simulink model "KTH_103002"  (Simulink 4.00)
settings: Solver=FixedStepDiscrete  StartTime=0.0  StopTime=5  RelTol=1e-3
values from neighbouring files (symbols this model uses):
  p2_1050 = [1.65 1.7 1.75 1.8 1.83 1.88 1.92 1.96 2.13 2.35 2.57 2.72 2.85 2.95]    [Comp1050_2.m]
  Pcomp_1050 = [690 790 880 1040 1160 1320 1580 1730 2970 5000 7960 9970 13200 16700]    [Comp1050_2.m]
  Qm_1050 = [2 2.5 3 4.5 5 6.5 8.5 10 20 35 55 65 85 100]    [Comp1050_2.m]
  T2_1050 = [99.2 103.5 107.2 110.7 111.8 112 111.7 100.4 116.5 131.5 136.4 147.4 149.6 155]    [Comp1050_2.m]
undefined symbols (not defined in the file or in its folder): conda, fan_cool, FC, fc_act, fc_blower_rec_H2, fc_blowera, fc_compressor, fc_condc, fc_coolstack, fc_current, fc_eqs, fc_evapcool, pump2, pump_cool, pump_re, radiator, vent
(part 2 of 2)

== system KTH_103002/PEM fuel cell system/Subsystem1/Anode init/Saturation pressure  anode humidifier ==
  note: Saturation pressure of water in the anode humidifier
      | NOTE: [bar]
      | Data from "Anlaggnings- och apparatteknik", Westerlund, T., Abo Akademi, Finland, 1998
  Anode humidifier temperature [C] : Constant  Value=FC.Lab.Temp.ah
  Anode humidifier temperature [C]1 : Constant  Value=FC.Lab.Temp.ah
  Constant : Constant  Value=11.78
  Constant1 : Constant  Value=99.64
  Constant2 : Constant  Value=230
  Math Function : Math  Operator=exp  OutputSignalType=auto
  Product : Product  Inputs=*/  Multiplication=Element-wise(.*)  SaturateOnIntegerOverflow=on
  Product1 : Product  Inputs=2  Multiplication=Element-wise(.*)  SaturateOnIntegerOverflow=on
  Sum : Sum  Inputs=|+-  SaturateOnIntegerOverflow=on
  Sum1 : Sum  Inputs=|++  SaturateOnIntegerOverflow=on
  psatah : Outport  Port=1
  tag scope: psatah=global
  wires:
  Anode humidifier temperature [C]/1 -> Sum/1
  Constant1/1 -> Sum/2
  Anode humidifier temperature [C]1/1 -> Sum1/1
  Constant2/1 -> Sum1/2
  Sum/1 -> Product/1
  Sum1/1 -> Product/2
  Constant/1 -> Product1/2
  Product/1 -> Product1/1
  Product1/1 -> Math Function/1
  Math Function/1 -> psatah/1, [psatah]

== system KTH_103002/PEM fuel cell system/Subsystem1/Anode init/Subsystem2 ==
  note: Activity of water vapor
  XWaI [-] : Inport  Port=1  LatchInput=off
  psatah [bar] : Inport  Port=2  LatchInput=off
  Constant : Constant  Value=FC.Lab.P.a
  Product : Product  Inputs=2  Multiplication=Element-wise(.*)  SaturateOnIntegerOverflow=on
  Product1 : Product  Inputs=*/  Multiplication=Element-wise(.*)  SaturateOnIntegerOverflow=on
  a : Outport  Port=1
  wires:
  XWaI [-]/1 -> Product/1
  Constant/1 -> Product/2
  Product/1 -> Product1/1
  psatah [bar]/1 -> Product1/2
  Product1/1 -> a/1

== system KTH_103002/PEM fuel cell system/Fuel cell stack, Heat Generation/Heat/Latent heat [W]/Heat of condensation ==
  note: Temperature in Celsius (C)
      | Tref=25 C
  note: 45.07E3 - 41.9*Tcell + 3.44E-3*Tcell^2 + 2.54E-6*Tcell^3 -8.98E-10*Tcell^4
  note: Heat of condensation [J/mol]
  Cell temperature [C] : Constant  Value=FC.Lab.Temp.cell
  Constant1 : Constant  Value=3.44E-3
  Constant2 : Constant  Value=45.07E3
  Constant3 : Constant  Value=41.9
  Constant4 : Constant  Value=2.54E-6
  Constant5 : Constant  Value=3
  Constant6 : Constant  Value=4
  Constant7 : Constant  Value=8.98E-10
  Display : Display
      settings: Format=short  Decimation=12
  Math Function : Math  Operator=square  OutputSignalType=auto
  Math Function1 : Math  Operator=pow  OutputSignalType=auto
  Math Function2 : Math  Operator=pow  OutputSignalType=auto
  Product{,1..3} (4 alike) : Product  Inputs=2  Multiplication=Element-wise(.*)  SaturateOnIntegerOverflow=on
  Sum : Sum  Inputs=|++  SaturateOnIntegerOverflow=on
  Sum1 : Sum  Inputs=|+-  SaturateOnIntegerOverflow=on
  Sum2 : Sum  Inputs=|++  SaturateOnIntegerOverflow=on
  Sum3 : Sum  Inputs=|+-  SaturateOnIntegerOverflow=on
  Hcond [J/mol] : Outport  Port=1
  wires:
  Constant3/1 -> Product/1
  Cell temperature [C]/1 -> Product/2, Math Function/1, Math Function1/1, Math Function2/1
  Product1/1 -> Sum/2
  Product/1 -> Sum1/2
  Constant2/1 -> Sum1/1
  Sum1/1 -> Sum/1
  Sum/1 -> Sum2/1
  Constant1/1 -> Product1/1
  Math Function/1 -> Product1/2
  Math Function1/1 -> Product2/2
  Constant4/1 -> Product2/1
  Product2/1 -> Sum2/2
  Sum2/1 -> Sum3/1
  Sum3/1 -> Hcond [J/mol]/1, Display/1
  Math Function2/1 -> Product3/2
  Product3/1 -> Sum3/2
  Constant7/1 -> Product3/1
  Constant5/1 -> Math Function1/2
  Constant6/1 -> Math Function2/2

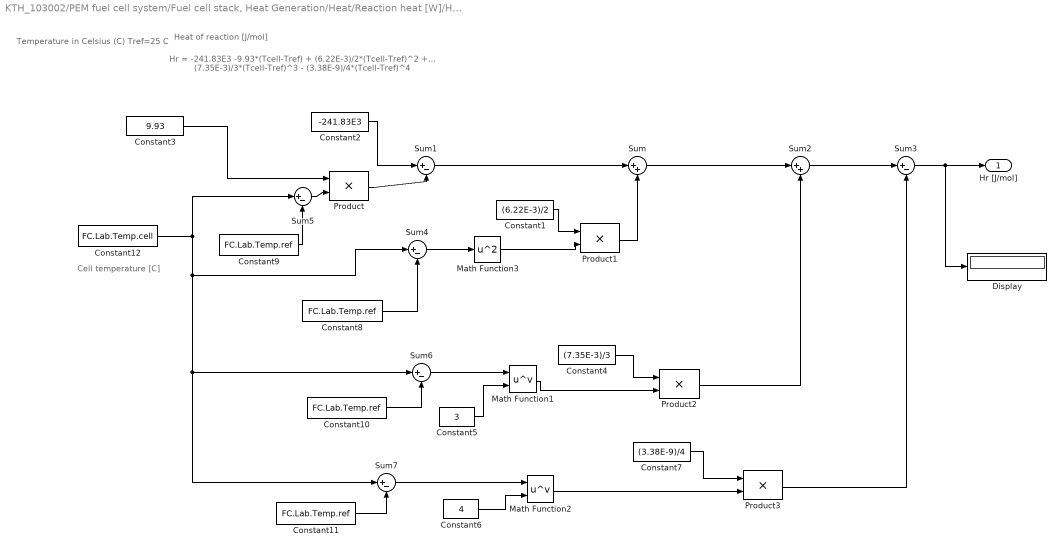
== system KTH_103002/PEM fuel cell system/Fuel cell stack, Heat Generation/Heat/Reaction heat [W]/Heat of reaction ==
  note: Temperature in Celsius (C)
      | Tref=25 C
  note: Hr = -241.83E3 -9.93*(Tcell-Tref) + (6.22E-3)/2*(Tcell-Tref)^2 +...
      |   (7.35E-3)/3*(Tcell-Tref)^3 - (3.38E-9)/4*(Tcell-Tref)^4
  note: Heat of reaction [J/mol]
  note: Cell temperature [C]
  Constant1 : Constant  Value=(6.22E-3)/2
  Constant{8..11} (4 alike) : Constant  Value=FC.Lab.Temp.ref
  Constant12 : Constant  Value=FC.Lab.Temp.cell
  Constant2 : Constant  Value=-241.83E3
  Constant3 : Constant  Value=9.93
  Constant4 : Constant  Value=(7.35E-3)/3
  Constant5 : Constant  Value=3
  Constant6 : Constant  Value=4
  Constant7 : Constant  Value=(3.38E-9)/4
  Display : Display
      settings: Format=short  Decimation=12
  Math Function1 : Math  Operator=pow  OutputSignalType=auto
  Math Function2 : Math  Operator=pow  OutputSignalType=auto
  Math Function3 : Math  Operator=square  OutputSignalType=auto
  Product{,1..3} (4 alike) : Product  Inputs=2  Multiplication=Element-wise(.*)  SaturateOnIntegerOverflow=on
  Sum : Sum  Inputs=|++  SaturateOnIntegerOverflow=on
  Sum{1,3..7} (6 alike) : Sum  Inputs=|+-  SaturateOnIntegerOverflow=on
  Sum2 : Sum  Inputs=|++  SaturateOnIntegerOverflow=on
  Hr [J/mol] : Outport  Port=1
  wires:
  Constant3/1 -> Product/1
  Product1/1 -> Sum/2
  Product/1 -> Sum1/2
  Constant2/1 -> Sum1/1
  Sum1/1 -> Sum/1
  Sum/1 -> Sum2/1
  Constant1/1 -> Product1/1
  Math Function1/1 -> Product2/2
  Constant4/1 -> Product2/1
  Product2/1 -> Sum2/2
  Sum2/1 -> Sum3/1
  Sum3/1 -> Hr [J/mol]/1, Display/1
  Math Function2/1 -> Product3/2
  Product3/1 -> Sum3/2
  Constant7/1 -> Product3/1
  Constant5/1 -> Math Function1/2
  Constant6/1 -> Math Function2/2
  Constant8/1 -> Sum4/2
  Sum5/1 -> Product/2
  Constant9/1 -> Sum5/2
  Sum4/1 -> Math Function3/1
  Math Function3/1 -> Product1/2
  Constant10/1 -> Sum6/2
  Sum6/1 -> Math Function1/1
  Constant11/1 -> Sum7/2
  Sum7/1 -> Math Function2/1
  Constant12/1 -> Sum5/1, Sum4/1, Sum6/1, Sum7/1

== system KTH_103002/PEM fuel cell system/Fuel cell stack, Heat Generation/Heat/Sensible heat [W]/Sensible heat in  ==
  note: Sensible heat in [W]
  note: Anode
  note: Cathode
  note: -------------------------------------------------------------------------------------------------------------------------------------------------------------------------------------------------------------------------------------------------------------------------------------------------------------------------------------------------------------------------------------------------------------------------------------------------------------------------------------------------------------------------------------------------------------------------------------------------------------------------------------------------------------------------------------------
  NinWa : Inport  Port=1  LatchInput=off
  NinHa : Inport  Port=2  LatchInput=off
  NinWc : Inport  Port=3  LatchInput=off
  NinO : Inport  Port=4  LatchInput=off
  NinN : Inport  Port=5  LatchInput=off
  "Enthalpy gaseous water, anode" : Subsystem
      settings: RTWFcnNameOpts=Auto  RTWFileNameOpts=Auto
  Enthalpy hydrogen in : Subsystem
      settings: RTWFcnNameOpts=Auto  RTWFileNameOpts=Auto
  Enthalpy nitrogen in : Subsystem
      settings: RTWFcnNameOpts=Auto  RTWFileNameOpts=Auto
  Enthalpy oxygen in : Subsystem
      settings: RTWFcnNameOpts=Auto  RTWFileNameOpts=Auto
  Product{,1..4} (5 alike) : Product  Inputs=2  Multiplication=Element-wise(.*)  SaturateOnIntegerOverflow=on
  Subsystem1 : Subsystem
      settings: RTWFcnNameOpts=Auto  RTWFileNameOpts=Auto
  Sum : Sum  Inputs=|++  SaturateOnIntegerOverflow=on
  Sum1 : Sum  Inputs=|++  SaturateOnIntegerOverflow=on
  Sum2 : Sum  Inputs=|++  SaturateOnIntegerOverflow=on
  sensina [W] : Outport  Port=1
  sensinc [W] : Outport  Port=2
  wires:
  NinHa/1 -> Product/1
  Enthalpy hydrogen in/1(h_Hin [J/mol]) -> Product/2
  Product/1 -> Sum/2
  NinWa/1 -> Product1/1
  Product1/1 -> Sum/1
  "Enthalpy gaseous water, anode"/1(h_Wgain [J/mol]) -> Product1/2
  NinWc/1 -> Product2/1
  Subsystem1/1(h_Wgcin [J/mol]) -> Product2/2
  Product2/1 -> Sum2/1
  NinO/1 -> Product3/1
  Enthalpy oxygen in/1(h_Oin [J/mol]) -> Product3/2
  Product3/1 -> Sum2/2
  Sum2/1 -> Sum1/1
  NinN/1 -> Product4/1
  Product4/1 -> Sum1/2
  Sum/1 -> sensina [W]/1
  Sum1/1 -> sensinc [W]/1
  Enthalpy nitrogen in/1(h_N [J/mol]) -> Product4/2

== system KTH_103002/PEM fuel cell system/Fuel cell stack, Heat Generation/Heat/Sensible heat [W]/Sensible heat out ==
  note: Sensible heat out [W]
  note: Anode
  note: Cathode
  note: -------------------------------------------------------------------------------------------------------------------------------------------------------------------------------------------------------------------------------------------------------------------------------------------------------------------------------------------------------------------------------------------------------------------------------------------------------------------------------------------------------------------------------------------------------------------------------------------------------------------------------------------------------------------------------------------
  note: Enthalpy gaseous water, cathode
  NoutWag : Inport  Port=1  LatchInput=off
  NoutHa : Inport  Port=2  LatchInput=off
  NoutWcg : Inport  Port=3  LatchInput=off
  NoutO : Inport  Port=4  LatchInput=off
  NoutN : Inport  Port=5  LatchInput=off
  NoutWcl : Inport  Port=6  LatchInput=off
  "Enthalpy gaseous water, anode" : Subsystem
      settings: RTWFcnNameOpts=Auto  RTWFileNameOpts=Auto
  Enthalpy hydrogen in : Subsystem
      settings: RTWFcnNameOpts=Auto  RTWFileNameOpts=Auto
  Enthalpy nitrogen out : Subsystem
      settings: RTWFcnNameOpts=Auto  RTWFileNameOpts=Auto
  Enthalpy oxygen out : Subsystem
      settings: RTWFcnNameOpts=Auto  RTWFileNameOpts=Auto
  Product{,1..5} (6 alike) : Product  Inputs=2  Multiplication=Element-wise(.*)  SaturateOnIntegerOverflow=on
  Subsystem1 : Subsystem
      settings: RTWFcnNameOpts=Auto  RTWFileNameOpts=Auto
  Subsystem2 : Subsystem
      settings: RTWFcnNameOpts=Auto  RTWFileNameOpts=Auto
  Sum{,1..3} (4 alike) : Sum  Inputs=|++  SaturateOnIntegerOverflow=on
  sensouta [W] : Outport  Port=1
  sensoutc [W] : Outport  Port=2
  wires:
  NoutHa/1 -> Product/1
  Enthalpy hydrogen in/1(h_Hout [J/mol]) -> Product/2
  Product/1 -> Sum/2
  NoutWag/1 -> Product1/1
  Product1/1 -> Sum/1
  "Enthalpy gaseous water, anode"/1(h_Wgaout [J/mol]) -> Product1/2
  NoutWcg/1 -> Product2/1
  Subsystem1/1(h_Wgcout [J/mol]) -> Product2/2
  Product2/1 -> Sum2/1
  NoutO/1 -> Product3/1
  Enthalpy oxygen out/1(h_Oout [J/mol]) -> Product3/2
  Product3/1 -> Sum2/2
  Sum2/1 -> Sum1/1
  NoutN/1 -> Product4/1
  Product4/1 -> Sum1/2
  Sum/1 -> sensouta [W]/1
  Enthalpy nitrogen out/1(h_N [J/mol]) -> Product4/2
  Sum1/1 -> Sum3/1
  Sum3/1 -> sensoutc [W]/1
  Subsystem2/1(h_Wl [J/mol]) -> Product5/2
  Product5/1 -> Sum3/2
  NoutWcl/1 -> Product5/1

== system KTH_103002/PEM fuel cell system/Humidifiers/Evapcooler/Ambient air/Humidity in air ==
  note: Humidity in air
  psat_air : Inport  Port=1  LatchInput=off
  Constant : Constant  Value=FC.Const.MW
  Constant1 : Constant  Value=FC.Lab.Stoich.RHo
  Constant2 : Constant  Value=FC.Const.Mair
  Constant3 : Constant  Value=FC.Lab.P.amb
  Constant4 : Constant  Value=100
  Constant6 : Constant  Value=FC.Lab.Stoich.RHo
  Constant7 : Constant  Value=100
  Display{,1..6} (7 alike) : Display
      settings: Format=short
  Product : Product  Inputs=*/  Multiplication=Element-wise(.*)  SaturateOnIntegerOverflow=on
  Product1 : Product  Inputs=*/  Multiplication=Element-wise(.*)  SaturateOnIntegerOverflow=on
  Product2 : Product  Inputs=3  Multiplication=Element-wise(.*)  SaturateOnIntegerOverflow=on
  Product3 : Product  Inputs=*/  Multiplication=Element-wise(.*)  SaturateOnIntegerOverflow=on
  Product4 : Product  Inputs=2  Multiplication=Element-wise(.*)  SaturateOnIntegerOverflow=on
  Product5 : Product  Inputs=/*  Multiplication=Element-wise(.*)  SaturateOnIntegerOverflow=on
  Sum : Sum  Inputs=|+-  SaturateOnIntegerOverflow=on
  wires:
  Constant/1 -> Product/1
  Constant2/1 -> Product/2
  Constant1/1 -> Product1/1
  Constant4/1 -> Product1/2
  psat_air/1 -> Product2/1, Product4/2
  Product1/1 -> Product2/3, Display4/1
  Product/1 -> Product2/2, Display3/1
  Constant6/1 -> Product3/1
  Constant7/1 -> Product3/2
  Constant3/1 -> Sum/1, Display6/1
  Product3/1 -> Sum/2
  Sum/1 -> Product4/1, Display5/1
  Product2/1 -> Product5/2, Display2/1
  Product4/1 -> Product5/1, Display1/1
  Product5/1 -> Display/1

== system KTH_103002/PEM fuel cell system/Humidifiers/Evapcooler/Ambient air/Saturation pressure ==
  note: Saturation pressure of water in the ambient air
      | NOTE: [bar]
      | Data from "Anlaggnings- och apparatteknik", Westerlund, T., Abo Akademi, Finland, 1998
  Ambient temperature [C] : Constant  Value=FC.Lab.Temp.amb
  Ambient temperature [C]1 : Constant  Value=FC.Lab.Temp.amb
  Constant : Constant  Value=11.78
  Constant1 : Constant  Value=99.64
  Constant2 : Constant  Value=230
  Display : Display
      settings: Format=short
  Math Function : Math  Operator=exp  OutputSignalType=auto
  Product : Product  Inputs=*/  Multiplication=Element-wise(.*)  SaturateOnIntegerOverflow=on
  Product1 : Product  Inputs=2  Multiplication=Element-wise(.*)  SaturateOnIntegerOverflow=on
  Sum : Sum  Inputs=|+-  SaturateOnIntegerOverflow=on
  Sum1 : Sum  Inputs=|++  SaturateOnIntegerOverflow=on
  psat_air : Outport  Port=1
  tag scope: psat_air=global
  wires:
  Ambient temperature [C]/1 -> Sum/1
  Constant1/1 -> Sum/2
  Ambient temperature [C]1/1 -> Sum1/1
  Constant2/1 -> Sum1/2
  Sum/1 -> Product/1
  Sum1/1 -> Product/2
  Constant/1 -> Product1/2
  Product/1 -> Product1/1
  Product1/1 -> Math Function/1
  Math Function/1 -> Display/1, psat_air/1, [psat_air]

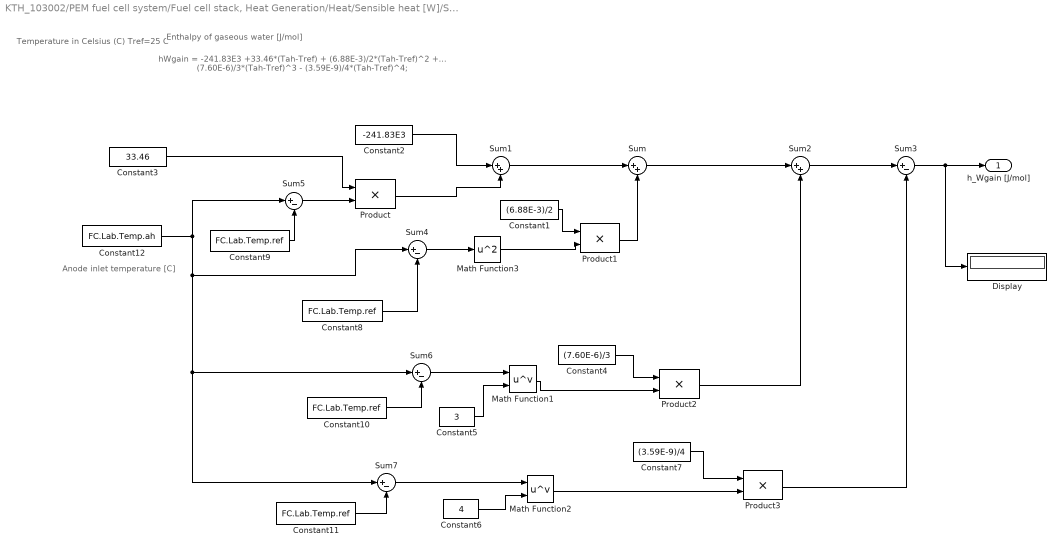
== system KTH_103002/PEM fuel cell system/Fuel cell stack, Heat Generation/Heat/Sensible heat [W]/Sensible heat in /Enthalpy gaseous water, anode ==
  note: Temperature in Celsius (C)
      | Tref=25 C
  note: hWgain = -241.83E3 +33.46*(Tah-Tref) + (6.88E-3)/2*(Tah-Tref)^2 +...
      |    (7.60E-6)/3*(Tah-Tref)^3 - (3.59E-9)/4*(Tah-Tref)^4;
  note: Enthalpy of gaseous water [J/mol]
  note: Anode inlet temperature [C]
  Constant1 : Constant  Value=(6.88E-3)/2
  Constant{8..11} (4 alike) : Constant  Value=FC.Lab.Temp.ref
  Constant12 : Constant  Value=FC.Lab.Temp.ah
  Constant2 : Constant  Value=-241.83E3
  Constant3 : Constant  Value=33.46
  Constant4 : Constant  Value=(7.60E-6)/3
  Constant5 : Constant  Value=3
  Constant6 : Constant  Value=4
  Constant7 : Constant  Value=(3.59E-9)/4
  Display : Display
      settings: Format=short  Decimation=12
  Math Function1 : Math  Operator=pow  OutputSignalType=auto
  Math Function2 : Math  Operator=pow  OutputSignalType=auto
  Math Function3 : Math  Operator=square  OutputSignalType=auto
  Product{,1..3} (4 alike) : Product  Inputs=2  Multiplication=Element-wise(.*)  SaturateOnIntegerOverflow=on
  Sum : Sum  Inputs=|++  SaturateOnIntegerOverflow=on
  Sum1 : Sum  Inputs=|++  SaturateOnIntegerOverflow=on
  Sum2 : Sum  Inputs=|++  SaturateOnIntegerOverflow=on
  Sum{3..7} (5 alike) : Sum  Inputs=|+-  SaturateOnIntegerOverflow=on
  h_Wgain [J/mol] : Outport  Port=1
  wires:
  Constant3/1 -> Product/1
  Product1/1 -> Sum/2
  Sum/1 -> Sum2/1
  Constant1/1 -> Product1/1
  Math Function1/1 -> Product2/2
  Constant4/1 -> Product2/1
  Product2/1 -> Sum2/2
  Sum2/1 -> Sum3/1
  Sum3/1 -> h_Wgain [J/mol]/1, Display/1
  Math Function2/1 -> Product3/2
  Product3/1 -> Sum3/2
  Constant7/1 -> Product3/1
  Constant5/1 -> Math Function1/2
  Constant6/1 -> Math Function2/2
  Constant8/1 -> Sum4/2
  Sum5/1 -> Product/2
  Constant9/1 -> Sum5/2
  Sum4/1 -> Math Function3/1
  Math Function3/1 -> Product1/2
  Constant10/1 -> Sum6/2
  Sum6/1 -> Math Function1/1
  Constant11/1 -> Sum7/2
  Sum7/1 -> Math Function2/1
  Constant12/1 -> Sum5/1, Sum4/1, Sum6/1, Sum7/1
  Product/1 -> Sum1/2
  Sum1/1 -> Sum/1
  Constant2/1 -> Sum1/1

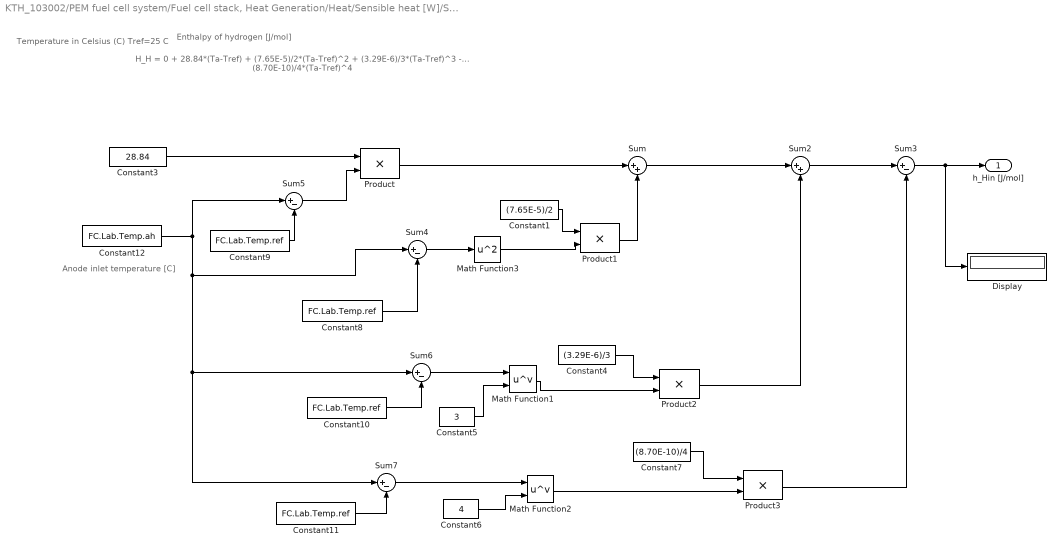
== system KTH_103002/PEM fuel cell system/Fuel cell stack, Heat Generation/Heat/Sensible heat [W]/Sensible heat in /Enthalpy hydrogen in ==
  note: Temperature in Celsius (C)
      | Tref=25 C
  note: H_H = 0 + 28.84*(Ta-Tref) + (7.65E-5)/2*(Ta-Tref)^2 + (3.29E-6)/3*(Ta-Tref)^3 -...
      |    (8.70E-10)/4*(Ta-Tref)^4
  note: Enthalpy of hydrogen [J/mol]
  note: Anode inlet temperature [C]
  Constant1 : Constant  Value=(7.65E-5)/2
  Constant{8..11} (4 alike) : Constant  Value=FC.Lab.Temp.ref
  Constant12 : Constant  Value=FC.Lab.Temp.ah
  Constant3 : Constant  Value=28.84
  Constant4 : Constant  Value=(3.29E-6)/3
  Constant5 : Constant  Value=3
  Constant6 : Constant  Value=4
  Constant7 : Constant  Value=(8.70E-10)/4
  Display : Display
      settings: Format=short  Decimation=12
  Math Function1 : Math  Operator=pow  OutputSignalType=auto
  Math Function2 : Math  Operator=pow  OutputSignalType=auto
  Math Function3 : Math  Operator=square  OutputSignalType=auto
  Product{,1..3} (4 alike) : Product  Inputs=2  Multiplication=Element-wise(.*)  SaturateOnIntegerOverflow=on
  Sum : Sum  Inputs=|++  SaturateOnIntegerOverflow=on
  Sum2 : Sum  Inputs=|++  SaturateOnIntegerOverflow=on
  Sum{3..7} (5 alike) : Sum  Inputs=|+-  SaturateOnIntegerOverflow=on
  h_Hin [J/mol] : Outport  Port=1
  wires:
  Constant3/1 -> Product/1
  Product1/1 -> Sum/2
  Sum/1 -> Sum2/1
  Constant1/1 -> Product1/1
  Math Function1/1 -> Product2/2
  Constant4/1 -> Product2/1
  Product2/1 -> Sum2/2
  Sum2/1 -> Sum3/1
  Sum3/1 -> h_Hin [J/mol]/1, Display/1
  Math Function2/1 -> Product3/2
  Product3/1 -> Sum3/2
  Constant7/1 -> Product3/1
  Constant5/1 -> Math Function1/2
  Constant6/1 -> Math Function2/2
  Constant8/1 -> Sum4/2
  Sum5/1 -> Product/2
  Constant9/1 -> Sum5/2
  Sum4/1 -> Math Function3/1
  Math Function3/1 -> Product1/2
  Constant10/1 -> Sum6/2
  Sum6/1 -> Math Function1/1
  Constant11/1 -> Sum7/2
  Sum7/1 -> Math Function2/1
  Constant12/1 -> Sum5/1, Sum4/1, Sum6/1, Sum7/1
  Product/1 -> Sum/1

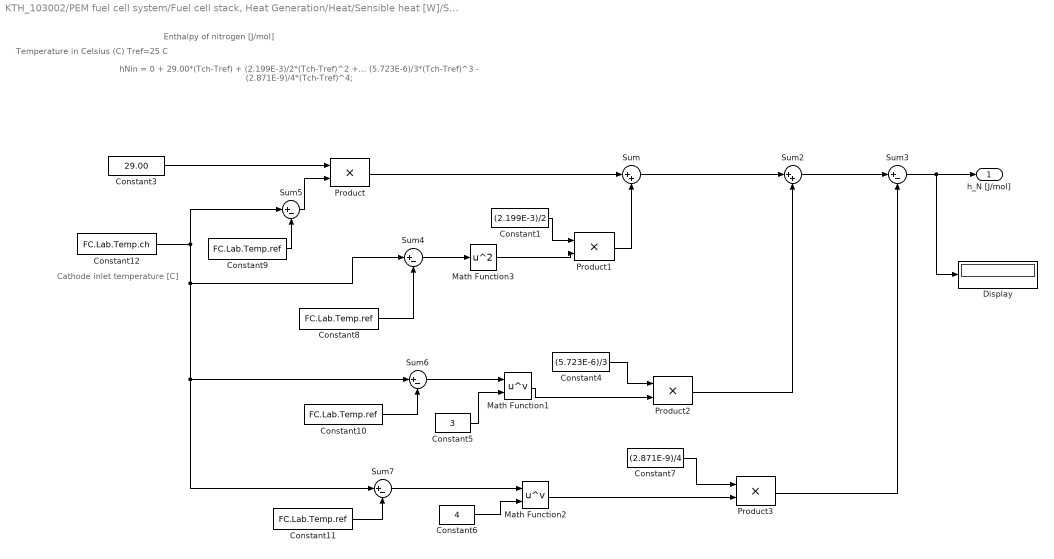
== system KTH_103002/PEM fuel cell system/Fuel cell stack, Heat Generation/Heat/Sensible heat [W]/Sensible heat in /Enthalpy nitrogen in ==
  note: Temperature in Celsius (C)
      | Tref=25 C
  note: hNin = 0 + 29.00*(Tch-Tref) + (2.199E-3)/2*(Tch-Tref)^2 +...
      |    (5.723E-6)/3*(Tch-Tref)^3 - (2.871E-9)/4*(Tch-Tref)^4;
  note: Enthalpy of nitrogen [J/mol]
  note: Cathode inlet temperature [C]
  Constant1 : Constant  Value=(2.199E-3)/2
  Constant{8..11} (4 alike) : Constant  Value=FC.Lab.Temp.ref
  Constant12 : Constant  Value=FC.Lab.Temp.ch
  Constant3 : Constant  Value=29.00
  Constant4 : Constant  Value=(5.723E-6)/3
  Constant5 : Constant  Value=3
  Constant6 : Constant  Value=4
  Constant7 : Constant  Value=(2.871E-9)/4
  Display : Display
      settings: Format=short  Decimation=12
  Math Function1 : Math  Operator=pow  OutputSignalType=auto
  Math Function2 : Math  Operator=pow  OutputSignalType=auto
  Math Function3 : Math  Operator=square  OutputSignalType=auto
  Product{,1..3} (4 alike) : Product  Inputs=2  Multiplication=Element-wise(.*)  SaturateOnIntegerOverflow=on
  Sum : Sum  Inputs=|++  SaturateOnIntegerOverflow=on
  Sum2 : Sum  Inputs=|++  SaturateOnIntegerOverflow=on
  Sum{3..7} (5 alike) : Sum  Inputs=|+-  SaturateOnIntegerOverflow=on
  h_N [J/mol] : Outport  Port=1
  wires:
  Constant3/1 -> Product/1
  Product1/1 -> Sum/2
  Product/1 -> Sum/1
  Sum/1 -> Sum2/1
  Constant1/1 -> Product1/1
  Math Function1/1 -> Product2/2
  Constant4/1 -> Product2/1
  Product2/1 -> Sum2/2
  Sum2/1 -> Sum3/1
  Sum3/1 -> h_N [J/mol]/1, Display/1
  Math Function2/1 -> Product3/2
  Product3/1 -> Sum3/2
  Constant7/1 -> Product3/1
  Constant5/1 -> Math Function1/2
  Constant6/1 -> Math Function2/2
  Constant8/1 -> Sum4/2
  Sum5/1 -> Product/2
  Constant9/1 -> Sum5/2
  Sum4/1 -> Math Function3/1
  Math Function3/1 -> Product1/2
  Constant10/1 -> Sum6/2
  Sum6/1 -> Math Function1/1
  Constant11/1 -> Sum7/2
  Sum7/1 -> Math Function2/1
  Constant12/1 -> Sum5/1, Sum4/1, Sum6/1, Sum7/1

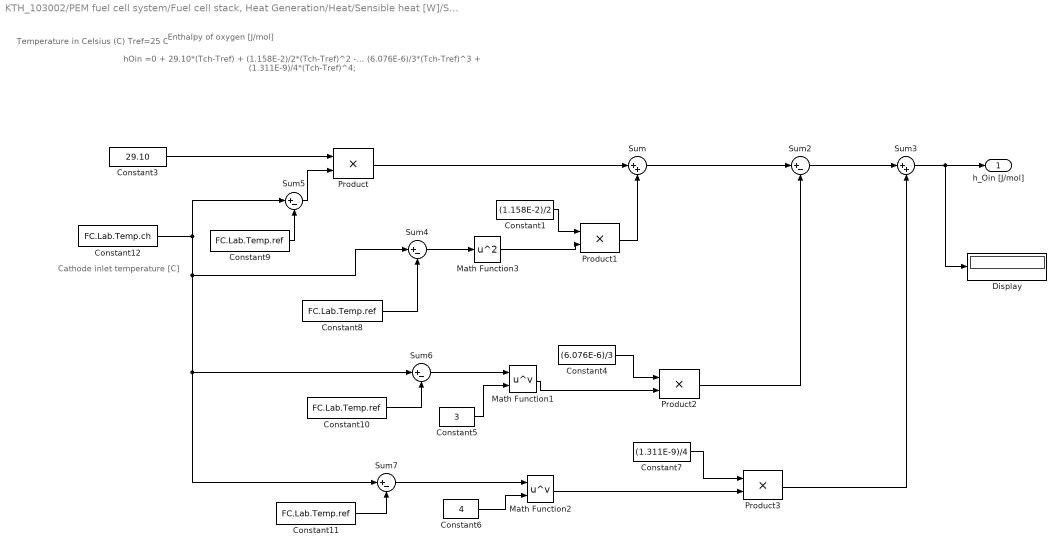
== system KTH_103002/PEM fuel cell system/Fuel cell stack, Heat Generation/Heat/Sensible heat [W]/Sensible heat in /Enthalpy oxygen in ==
  note: Temperature in Celsius (C)
      | Tref=25 C
  note: hOin =0 + 29.10*(Tch-Tref) + (1.158E-2)/2*(Tch-Tref)^2 -...
      |    (6.076E-6)/3*(Tch-Tref)^3 + (1.311E-9)/4*(Tch-Tref)^4;
  note: Enthalpy of oxygen [J/mol]
  note: Cathode inlet temperature [C]
  Constant1 : Constant  Value=(1.158E-2)/2
  Constant{8..11} (4 alike) : Constant  Value=FC.Lab.Temp.ref
  Constant12 : Constant  Value=FC.Lab.Temp.ch
  Constant3 : Constant  Value=29.10
  Constant4 : Constant  Value=(6.076E-6)/3
  Constant5 : Constant  Value=3
  Constant6 : Constant  Value=4
  Constant7 : Constant  Value=(1.311E-9)/4
  Display : Display
      settings: Format=short  Decimation=12
  Math Function1 : Math  Operator=pow  OutputSignalType=auto
  Math Function2 : Math  Operator=pow  OutputSignalType=auto
  Math Function3 : Math  Operator=square  OutputSignalType=auto
  Product{,1..3} (4 alike) : Product  Inputs=2  Multiplication=Element-wise(.*)  SaturateOnIntegerOverflow=on
  Sum : Sum  Inputs=|++  SaturateOnIntegerOverflow=on
  Sum{2,4..7} (5 alike) : Sum  Inputs=|+-  SaturateOnIntegerOverflow=on
  Sum3 : Sum  Inputs=|++  SaturateOnIntegerOverflow=on
  h_Oin [J/mol] : Outport  Port=1
  wires:
  Constant3/1 -> Product/1
  Product1/1 -> Sum/2
  Product/1 -> Sum/1
  Sum/1 -> Sum2/1
  Constant1/1 -> Product1/1
  Math Function1/1 -> Product2/2
  Constant4/1 -> Product2/1
  Product2/1 -> Sum2/2
  Sum2/1 -> Sum3/1
  Sum3/1 -> h_Oin [J/mol]/1, Display/1
  Math Function2/1 -> Product3/2
  Product3/1 -> Sum3/2
  Constant7/1 -> Product3/1
  Constant5/1 -> Math Function1/2
  Constant6/1 -> Math Function2/2
  Constant8/1 -> Sum4/2
  Sum5/1 -> Product/2
  Constant9/1 -> Sum5/2
  Sum4/1 -> Math Function3/1
  Math Function3/1 -> Product1/2
  Constant10/1 -> Sum6/2
  Sum6/1 -> Math Function1/1
  Constant11/1 -> Sum7/2
  Sum7/1 -> Math Function2/1
  Constant12/1 -> Sum5/1, Sum4/1, Sum6/1, Sum7/1

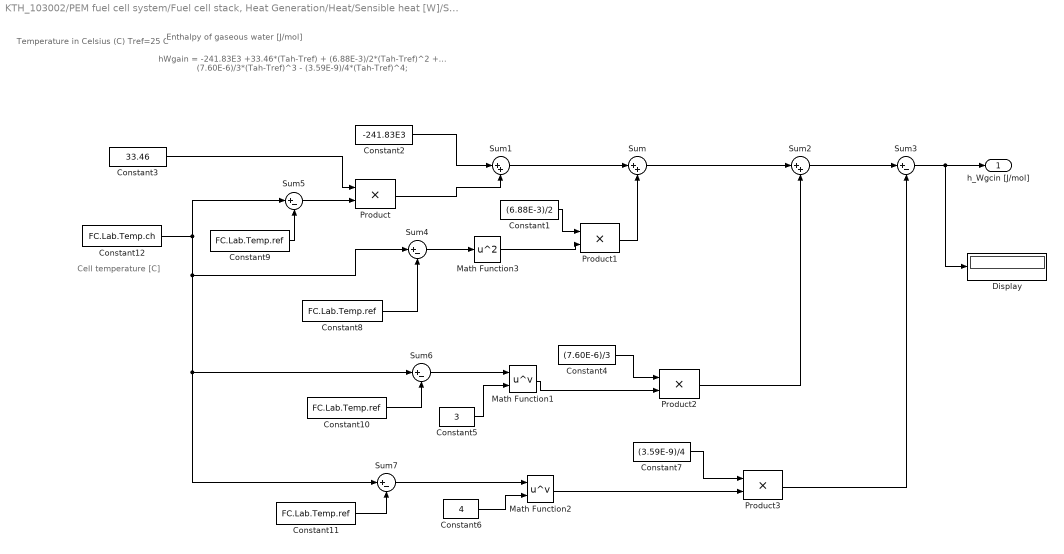
== system KTH_103002/PEM fuel cell system/Fuel cell stack, Heat Generation/Heat/Sensible heat [W]/Sensible heat in /Subsystem1 ==
  note: Temperature in Celsius (C)
      | Tref=25 C
  note: hWgain = -241.83E3 +33.46*(Tah-Tref) + (6.88E-3)/2*(Tah-Tref)^2 +...
      |    (7.60E-6)/3*(Tah-Tref)^3 - (3.59E-9)/4*(Tah-Tref)^4;
  note: Enthalpy of gaseous water [J/mol]
  note: Cell temperature [C]
  Constant1 : Constant  Value=(6.88E-3)/2
  Constant{8..11} (4 alike) : Constant  Value=FC.Lab.Temp.ref
  Constant12 : Constant  Value=FC.Lab.Temp.ch
  Constant2 : Constant  Value=-241.83E3
  Constant3 : Constant  Value=33.46
  Constant4 : Constant  Value=(7.60E-6)/3
  Constant5 : Constant  Value=3
  Constant6 : Constant  Value=4
  Constant7 : Constant  Value=(3.59E-9)/4
  Display : Display
      settings: Format=short  Decimation=12
  Math Function1 : Math  Operator=pow  OutputSignalType=auto
  Math Function2 : Math  Operator=pow  OutputSignalType=auto
  Math Function3 : Math  Operator=square  OutputSignalType=auto
  Product{,1..3} (4 alike) : Product  Inputs=2  Multiplication=Element-wise(.*)  SaturateOnIntegerOverflow=on
  Sum : Sum  Inputs=|++  SaturateOnIntegerOverflow=on
  Sum1 : Sum  Inputs=|++  SaturateOnIntegerOverflow=on
  Sum2 : Sum  Inputs=|++  SaturateOnIntegerOverflow=on
  Sum{3..7} (5 alike) : Sum  Inputs=|+-  SaturateOnIntegerOverflow=on
  h_Wgcin [J/mol] : Outport  Port=1
  wires:
  Constant3/1 -> Product/1
  Product1/1 -> Sum/2
  Sum/1 -> Sum2/1
  Constant1/1 -> Product1/1
  Math Function1/1 -> Product2/2
  Constant4/1 -> Product2/1
  Product2/1 -> Sum2/2
  Sum2/1 -> Sum3/1
  Sum3/1 -> h_Wgcin [J/mol]/1, Display/1
  Math Function2/1 -> Product3/2
  Product3/1 -> Sum3/2
  Constant7/1 -> Product3/1
  Constant5/1 -> Math Function1/2
  Constant6/1 -> Math Function2/2
  Constant8/1 -> Sum4/2
  Sum5/1 -> Product/2
  Constant9/1 -> Sum5/2
  Sum4/1 -> Math Function3/1
  Math Function3/1 -> Product1/2
  Constant10/1 -> Sum6/2
  Sum6/1 -> Math Function1/1
  Constant11/1 -> Sum7/2
  Sum7/1 -> Math Function2/1
  Constant12/1 -> Sum5/1, Sum4/1, Sum6/1, Sum7/1
  Product/1 -> Sum1/2
  Sum1/1 -> Sum/1
  Constant2/1 -> Sum1/1

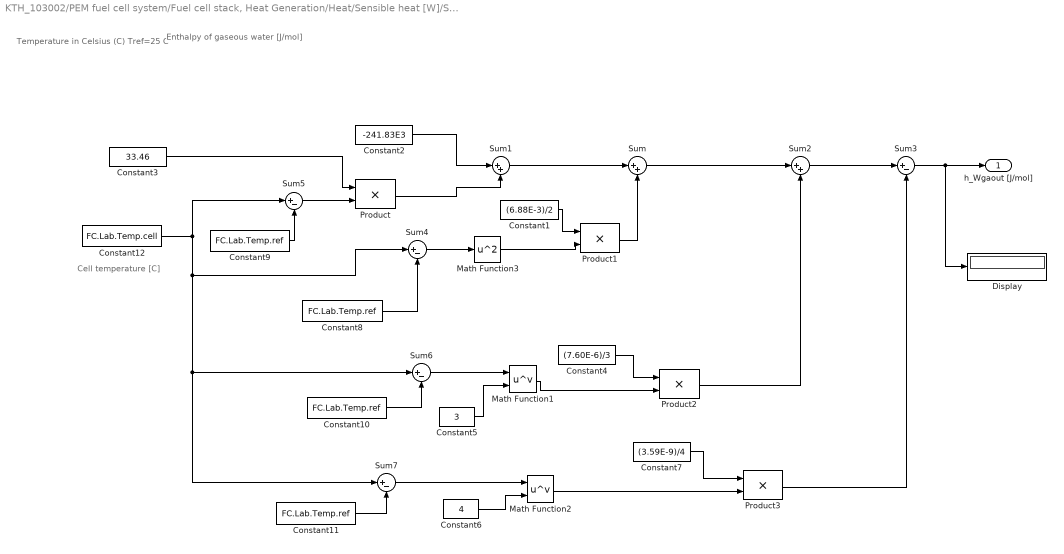
== system KTH_103002/PEM fuel cell system/Fuel cell stack, Heat Generation/Heat/Sensible heat [W]/Sensible heat out/Enthalpy gaseous water, anode ==
  note: Temperature in Celsius (C)
      | Tref=25 C
  note: Enthalpy of gaseous water [J/mol]
  note: Cell temperature [C]
  Constant1 : Constant  Value=(6.88E-3)/2
  Constant{8..11} (4 alike) : Constant  Value=FC.Lab.Temp.ref
  Constant12 : Constant  Value=FC.Lab.Temp.cell
  Constant2 : Constant  Value=-241.83E3
  Constant3 : Constant  Value=33.46
  Constant4 : Constant  Value=(7.60E-6)/3
  Constant5 : Constant  Value=3
  Constant6 : Constant  Value=4
  Constant7 : Constant  Value=(3.59E-9)/4
  Display : Display
      settings: Format=short  Decimation=12
  Math Function1 : Math  Operator=pow  OutputSignalType=auto
  Math Function2 : Math  Operator=pow  OutputSignalType=auto
  Math Function3 : Math  Operator=square  OutputSignalType=auto
  Product{,1..3} (4 alike) : Product  Inputs=2  Multiplication=Element-wise(.*)  SaturateOnIntegerOverflow=on
  Sum : Sum  Inputs=|++  SaturateOnIntegerOverflow=on
  Sum1 : Sum  Inputs=|++  SaturateOnIntegerOverflow=on
  Sum2 : Sum  Inputs=|++  SaturateOnIntegerOverflow=on
  Sum{3..7} (5 alike) : Sum  Inputs=|+-  SaturateOnIntegerOverflow=on
  h_Wgaout [J/mol] : Outport  Port=1
  wires:
  Constant3/1 -> Product/1
  Product1/1 -> Sum/2
  Sum/1 -> Sum2/1
  Constant1/1 -> Product1/1
  Math Function1/1 -> Product2/2
  Constant4/1 -> Product2/1
  Product2/1 -> Sum2/2
  Sum2/1 -> Sum3/1
  Sum3/1 -> h_Wgaout [J/mol]/1, Display/1
  Math Function2/1 -> Product3/2
  Product3/1 -> Sum3/2
  Constant7/1 -> Product3/1
  Constant5/1 -> Math Function1/2
  Constant6/1 -> Math Function2/2
  Constant8/1 -> Sum4/2
  Sum5/1 -> Product/2
  Constant9/1 -> Sum5/2
  Sum4/1 -> Math Function3/1
  Math Function3/1 -> Product1/2
  Constant10/1 -> Sum6/2
  Sum6/1 -> Math Function1/1
  Constant11/1 -> Sum7/2
  Sum7/1 -> Math Function2/1
  Constant12/1 -> Sum5/1, Sum4/1, Sum6/1, Sum7/1
  Product/1 -> Sum1/2
  Sum1/1 -> Sum/1
  Constant2/1 -> Sum1/1

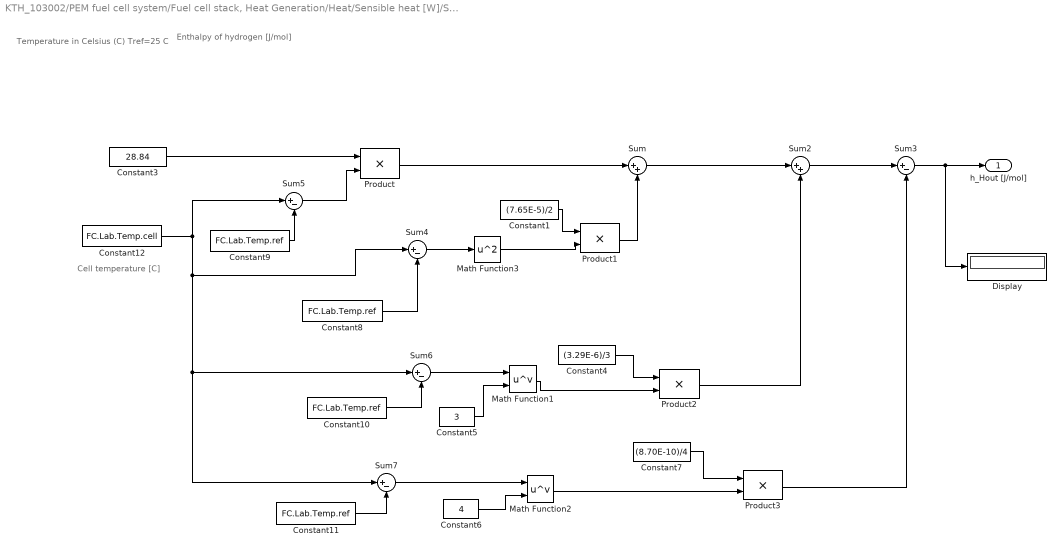
== system KTH_103002/PEM fuel cell system/Fuel cell stack, Heat Generation/Heat/Sensible heat [W]/Sensible heat out/Enthalpy hydrogen in ==
  note: Temperature in Celsius (C)
      | Tref=25 C
  note: Enthalpy of hydrogen [J/mol]
  note: Cell temperature [C]
  Constant1 : Constant  Value=(7.65E-5)/2
  Constant{8..11} (4 alike) : Constant  Value=FC.Lab.Temp.ref
  Constant12 : Constant  Value=FC.Lab.Temp.cell
  Constant3 : Constant  Value=28.84
  Constant4 : Constant  Value=(3.29E-6)/3
  Constant5 : Constant  Value=3
  Constant6 : Constant  Value=4
  Constant7 : Constant  Value=(8.70E-10)/4
  Display : Display
      settings: Format=short  Decimation=12
  Math Function1 : Math  Operator=pow  OutputSignalType=auto
  Math Function2 : Math  Operator=pow  OutputSignalType=auto
  Math Function3 : Math  Operator=square  OutputSignalType=auto
  Product{,1..3} (4 alike) : Product  Inputs=2  Multiplication=Element-wise(.*)  SaturateOnIntegerOverflow=on
  Sum : Sum  Inputs=|++  SaturateOnIntegerOverflow=on
  Sum2 : Sum  Inputs=|++  SaturateOnIntegerOverflow=on
  Sum{3..7} (5 alike) : Sum  Inputs=|+-  SaturateOnIntegerOverflow=on
  h_Hout [J/mol] : Outport  Port=1
  wires:
  Constant3/1 -> Product/1
  Product1/1 -> Sum/2
  Sum/1 -> Sum2/1
  Constant1/1 -> Product1/1
  Math Function1/1 -> Product2/2
  Constant4/1 -> Product2/1
  Product2/1 -> Sum2/2
  Sum2/1 -> Sum3/1
  Sum3/1 -> h_Hout [J/mol]/1, Display/1
  Math Function2/1 -> Product3/2
  Product3/1 -> Sum3/2
  Constant7/1 -> Product3/1
  Constant5/1 -> Math Function1/2
  Constant6/1 -> Math Function2/2
  Constant8/1 -> Sum4/2
  Sum5/1 -> Product/2
  Constant9/1 -> Sum5/2
  Sum4/1 -> Math Function3/1
  Math Function3/1 -> Product1/2
  Constant10/1 -> Sum6/2
  Sum6/1 -> Math Function1/1
  Constant11/1 -> Sum7/2
  Sum7/1 -> Math Function2/1
  Constant12/1 -> Sum5/1, Sum4/1, Sum6/1, Sum7/1
  Product/1 -> Sum/1

== system KTH_103002/PEM fuel cell system/Fuel cell stack, Heat Generation/Heat/Sensible heat [W]/Sensible heat out/Enthalpy nitrogen out ==
  note: Temperature in Celsius (C)
      | Tref=25 C
  note: Enthalpy of nitrogen [J/mol]
  note: Cell temperature [C]
  Constant1 : Constant  Value=(2.199E-3)/2
  Constant{8..11} (4 alike) : Constant  Value=FC.Lab.Temp.ref
  Constant12 : Constant  Value=FC.Lab.Temp.cell
  Constant3 : Constant  Value=29.00
  Constant4 : Constant  Value=(5.723E-6)/3
  Constant5 : Constant  Value=3
  Constant6 : Constant  Value=4
  Constant7 : Constant  Value=(2.871E-9)/4
  Display : Display
      settings: Format=short  Decimation=12
  Math Function1 : Math  Operator=pow  OutputSignalType=auto
  Math Function2 : Math  Operator=pow  OutputSignalType=auto
  Math Function3 : Math  Operator=square  OutputSignalType=auto
  Product{,1..3} (4 alike) : Product  Inputs=2  Multiplication=Element-wise(.*)  SaturateOnIntegerOverflow=on
  Sum : Sum  Inputs=|++  SaturateOnIntegerOverflow=on
  Sum2 : Sum  Inputs=|++  SaturateOnIntegerOverflow=on
  Sum{3..7} (5 alike) : Sum  Inputs=|+-  SaturateOnIntegerOverflow=on
  h_N [J/mol] : Outport  Port=1
  wires:
  Constant3/1 -> Product/1
  Product1/1 -> Sum/2
  Product/1 -> Sum/1
  Sum/1 -> Sum2/1
  Constant1/1 -> Product1/1
  Math Function1/1 -> Product2/2
  Constant4/1 -> Product2/1
  Product2/1 -> Sum2/2
  Sum2/1 -> Sum3/1
  Sum3/1 -> h_N [J/mol]/1, Display/1
  Math Function2/1 -> Product3/2
  Product3/1 -> Sum3/2
  Constant7/1 -> Product3/1
  Constant5/1 -> Math Function1/2
  Constant6/1 -> Math Function2/2
  Constant8/1 -> Sum4/2
  Sum5/1 -> Product/2
  Constant9/1 -> Sum5/2
  Sum4/1 -> Math Function3/1
  Math Function3/1 -> Product1/2
  Constant10/1 -> Sum6/2
  Sum6/1 -> Math Function1/1
  Constant11/1 -> Sum7/2
  Sum7/1 -> Math Function2/1
  Constant12/1 -> Sum5/1, Sum4/1, Sum6/1, Sum7/1

== system KTH_103002/PEM fuel cell system/Fuel cell stack, Heat Generation/Heat/Sensible heat [W]/Sensible heat out/Enthalpy oxygen out ==
  note: Temperature in Celsius (C)
      | Tref=25 C
  note: Enthalpy of oxygen [J/mol]
  note: Cell temperature [C]
  Constant1 : Constant  Value=(1.158E-2)/2
  Constant{8..11} (4 alike) : Constant  Value=FC.Lab.Temp.ref
  Constant12 : Constant  Value=FC.Lab.Temp.cell
  Constant3 : Constant  Value=29.10
  Constant4 : Constant  Value=(6.076E-6)/3
  Constant5 : Constant  Value=3
  Constant6 : Constant  Value=4
  Constant7 : Constant  Value=(1.311E-9)/4
  Display : Display
      settings: Format=short  Decimation=12
  Math Function1 : Math  Operator=pow  OutputSignalType=auto
  Math Function2 : Math  Operator=pow  OutputSignalType=auto
  Math Function3 : Math  Operator=square  OutputSignalType=auto
  Product{,1..3} (4 alike) : Product  Inputs=2  Multiplication=Element-wise(.*)  SaturateOnIntegerOverflow=on
  Sum : Sum  Inputs=|++  SaturateOnIntegerOverflow=on
  Sum{2,4..7} (5 alike) : Sum  Inputs=|+-  SaturateOnIntegerOverflow=on
  Sum3 : Sum  Inputs=|++  SaturateOnIntegerOverflow=on
  h_Oout [J/mol] : Outport  Port=1
  wires:
  Constant3/1 -> Product/1
  Product1/1 -> Sum/2
  Product/1 -> Sum/1
  Sum/1 -> Sum2/1
  Constant1/1 -> Product1/1
  Math Function1/1 -> Product2/2
  Constant4/1 -> Product2/1
  Product2/1 -> Sum2/2
  Sum2/1 -> Sum3/1
  Sum3/1 -> h_Oout [J/mol]/1, Display/1
  Math Function2/1 -> Product3/2
  Product3/1 -> Sum3/2
  Constant7/1 -> Product3/1
  Constant5/1 -> Math Function1/2
  Constant6/1 -> Math Function2/2
  Constant8/1 -> Sum4/2
  Sum5/1 -> Product/2
  Constant9/1 -> Sum5/2
  Sum4/1 -> Math Function3/1
  Math Function3/1 -> Product1/2
  Constant10/1 -> Sum6/2
  Sum6/1 -> Math Function1/1
  Constant11/1 -> Sum7/2
  Sum7/1 -> Math Function2/1
  Constant12/1 -> Sum5/1, Sum4/1, Sum6/1, Sum7/1

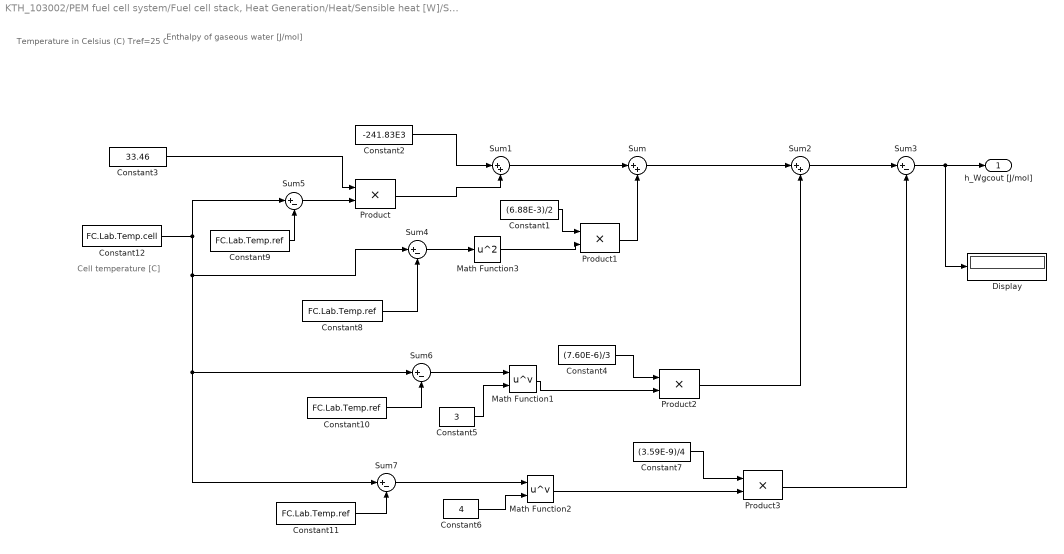
== system KTH_103002/PEM fuel cell system/Fuel cell stack, Heat Generation/Heat/Sensible heat [W]/Sensible heat out/Subsystem1 ==
  note: Temperature in Celsius (C)
      | Tref=25 C
  note: Enthalpy of gaseous water [J/mol]
  note: Cell temperature [C]
  Constant1 : Constant  Value=(6.88E-3)/2
  Constant{8..11} (4 alike) : Constant  Value=FC.Lab.Temp.ref
  Constant12 : Constant  Value=FC.Lab.Temp.cell
  Constant2 : Constant  Value=-241.83E3
  Constant3 : Constant  Value=33.46
  Constant4 : Constant  Value=(7.60E-6)/3
  Constant5 : Constant  Value=3
  Constant6 : Constant  Value=4
  Constant7 : Constant  Value=(3.59E-9)/4
  Display : Display
      settings: Format=short  Decimation=12
  Math Function1 : Math  Operator=pow  OutputSignalType=auto
  Math Function2 : Math  Operator=pow  OutputSignalType=auto
  Math Function3 : Math  Operator=square  OutputSignalType=auto
  Product{,1..3} (4 alike) : Product  Inputs=2  Multiplication=Element-wise(.*)  SaturateOnIntegerOverflow=on
  Sum : Sum  Inputs=|++  SaturateOnIntegerOverflow=on
  Sum1 : Sum  Inputs=|++  SaturateOnIntegerOverflow=on
  Sum2 : Sum  Inputs=|++  SaturateOnIntegerOverflow=on
  Sum{3..7} (5 alike) : Sum  Inputs=|+-  SaturateOnIntegerOverflow=on
  h_Wgcout [J/mol] : Outport  Port=1
  wires:
  Constant3/1 -> Product/1
  Product1/1 -> Sum/2
  Sum/1 -> Sum2/1
  Constant1/1 -> Product1/1
  Math Function1/1 -> Product2/2
  Constant4/1 -> Product2/1
  Product2/1 -> Sum2/2
  Sum2/1 -> Sum3/1
  Sum3/1 -> h_Wgcout [J/mol]/1, Display/1
  Math Function2/1 -> Product3/2
  Product3/1 -> Sum3/2
  Constant7/1 -> Product3/1
  Constant5/1 -> Math Function1/2
  Constant6/1 -> Math Function2/2
  Constant8/1 -> Sum4/2
  Sum5/1 -> Product/2
  Constant9/1 -> Sum5/2
  Sum4/1 -> Math Function3/1
  Math Function3/1 -> Product1/2
  Constant10/1 -> Sum6/2
  Sum6/1 -> Math Function1/1
  Constant11/1 -> Sum7/2
  Sum7/1 -> Math Function2/1
  Constant12/1 -> Sum5/1, Sum4/1, Sum6/1, Sum7/1
  Product/1 -> Sum1/2
  Sum1/1 -> Sum/1
  Constant2/1 -> Sum1/1

== system KTH_103002/PEM fuel cell system/Fuel cell stack, Heat Generation/Heat/Sensible heat [W]/Sensible heat out/Subsystem2 ==
  note: Temperature in Celsius (C)
      | Tref=25 C
  note: HWl = -285.84E3 + 75.38*(Tcell-Tref)
  note: Enthalpy of liquid water [J/mol]
  note: Cell temperature [C]
  Constant12 : Constant  Value=FC.Lab.Temp.cell
  Constant2 : Constant  Value=-285.84E3
  Constant3 : Constant  Value=75.38
  Constant9 : Constant  Value=FC.Lab.Temp.ref
  Display : Display
      settings: Format=short  Decimation=12
  Product : Product  Inputs=2  Multiplication=Element-wise(.*)  SaturateOnIntegerOverflow=on
  Sum1 : Sum  Inputs=|++  SaturateOnIntegerOverflow=on
  Sum5 : Sum  Inputs=|+-  SaturateOnIntegerOverflow=on
  h_Wl [J/mol] : Outport  Port=1
  wires:
  Constant3/1 -> Product/1
  Sum5/1 -> Product/2
  Constant9/1 -> Sum5/2
  Constant12/1 -> Sum5/1
  Product/1 -> Sum1/2
  Constant2/1 -> Sum1/1
  Sum1/1 -> h_Wl [J/mol]/1, Display/1
